simulink model "B733_JSB_R17a"  (R2017a)
settings: Solver=VariableStepAuto  StartTime=0.0  StopTime=simtime  RelTol=1e-3
undefined symbols (not defined in the file): engineCount, engineLUT, Tmil, xu
libraries: aerolibanim x1, aerolibatmos2 x1, aerolibgravity2 x1
settings Model: Creator=Can Bekar  LastModifiedBy=Can Bekar
settings DataIOCC: ExternalInput=usignal  InitialState=xu  LoadExternalInput=on  LoadInitialState=on  SaveFormat=Array

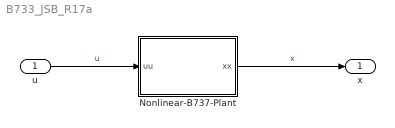
== system B733_JSB_R17a ==
  u : Inport
  Nonlinear-B737-Plant : Subsystem
  x : Outport
  wires:
  u/1 -> Nonlinear-B737-Plant/1(uu)  "u"
  Nonlinear-B737-Plant/1(xx) -> x/1  "x"

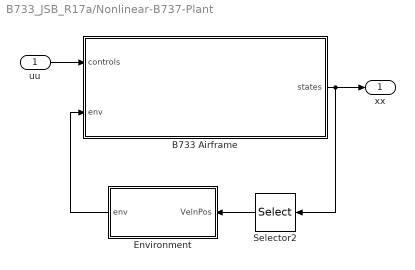
== system B733_JSB_R17a/Nonlinear-B737-Plant ==
  uu : Inport
  B733 Airframe : Subsystem
      mask Display: image('300Large.png');
  Environment : Subsystem
      mask Display: image('ww15mgh2.jpg');
  Selector2 : Selector  InputPortWidth=12  IndexOptions=Index vector (dialog)  Indices=[1 10 11 12]  OutputSizes=1
  xx : Outport
  wires:
  uu/1 -> B733 Airframe/1(controls)
  B733 Airframe/1(states) -> xx/1, Selector2/1
  Selector2/1 -> Environment/1(VelnPos)
  Environment/1(env) -> B733 Airframe/2(env)

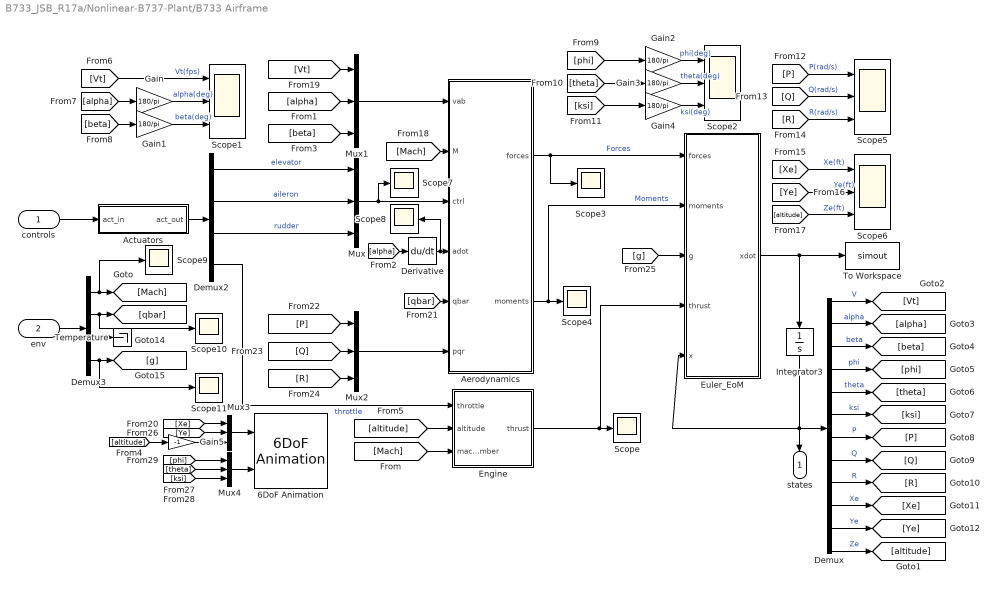
== system B733_JSB_R17a/Nonlinear-B737-Plant/B733 Airframe ==
  controls : Inport
  env : Inport  Port=2
  6DoF Animation : aerolibanim/6DoF Animation  u1=[0 100000 -100000 100000 0 35000]  u2=1  u3=15000.0  u4=[0 0 0]  u5=Fixed position  u6=[100000 20000 -xu(12)]  u7=30  u8=on
      settings: SourceProductName=Aerospace Blockset
  Actuators : Subsystem
  Aerodynamics : MATLAB Function  TreatAsAtomicUnit=on
  Demux : Demux  Outputs=12
  Demux2 : Demux
  Demux3 : Demux
  Derivative : Derivative
  Engine : Subsystem
  Euler_EoM : MATLAB Function  TreatAsAtomicUnit=on
  Gain{,1..4} (5 alike) : Gain  Gain=180/pi
  Gain5 : Gain  Gain=-1
  Integrator3 : Integrator  InitialCondition=xu
  Mux{,1..4} (5 alike) : Mux  Inputs=3
  Scope{,3..4,7..11} (8 alike) : Scope
  Scope{1..2,5..6} (4 alike) : Scope  NumInputPorts=3
  Temperature : Terminator
  To Workspace : ToWorkspace  VariableName=simout  SampleTime=-1
  states : Outport
  wires:
  Actuators/1(act_out) -> Demux2/1
  [Mach] -> Engine/3(mach_number)
  Integrator3/1 -> Euler_EoM/5(x), states/1, Demux/1
  Demux/1 -> [Vt]  "V"
  Demux/3 -> [beta]  "beta"
  [alpha] -> Derivative/1
  [altitude] -> Engine/2(altitude)
  Demux/12 -> [altitude]  "Ze"
  [Vt] -> Scope1/1  "Vt(fps)"
  Demux/11 -> [Ye]  "Ye"
  Demux/10 -> [Xe]  "Xe"
  Demux/9 -> [R]  "R"
  Demux/8 -> [Q]  "Q"
  Demux/7 -> [P]  "P"
  Demux/6 -> [ksi]  "ksi"
  Demux/5 -> [theta]  "theta"
  Demux/4 -> [phi]  "phi"
  [theta] -> Gain3/1
  [phi] -> Gain2/1
  [ksi] -> Gain4/1
  [R] -> Scope5/3  "R(rad/s)"
  [Q] -> Scope5/2  "Q(rad/s)"
  [P] -> Scope5/1  "P(rad/s)"
  [Xe] -> Scope6/1  "Xe(ft)"
  [altitude] -> Scope6/3  "Ze(ft)"
  [Ye] -> Scope6/2  "Ye(ft)"
  Engine/1(thrust) -> Euler_EoM/4(thrust), Scope/1
  [Mach] -> Aerodynamics/2(M)
  Demux2/1 -> Mux/1  "elevator"
  Demux2/2 -> Mux/2  "aileron"
  Demux2/3 -> Mux/3  "rudder"
  [qbar] -> Aerodynamics/5(qbar)
  Gain/1 -> Scope1/2  "alpha(deg)"
  [alpha] -> Gain/1
  [beta] -> Gain1/1
  Gain1/1 -> Scope1/3  "beta(deg)"
  Aerodynamics/1(forces) -> Scope3/1, Euler_EoM/1(forces)  "Forces"
  Aerodynamics/2(moments) -> Euler_EoM/2(moments), Scope4/1  "Moments"
  [g] -> Euler_EoM/3(g)
  Demux/2 -> [alpha]  "alpha"
  Euler_EoM/1(xdot) -> To Workspace/1, Integrator3/1
  Gain2/1 -> Scope2/1  "phi(deg)"
  Gain3/1 -> Scope2/2  "theta(deg)"
  Gain4/1 -> Scope2/3  "ksi(deg)"
  controls/1 -> Actuators/1(act_in)
  Demux2/4 -> Engine/1(throttle)  "throttle"
  env/1 -> Demux3/1
  Demux3/1 -> Scope9/1, [Mach]
  Demux3/2 -> Scope10/1, [qbar]
  Demux3/3 -> Temperature/1
  Demux3/4 -> Scope11/1, [g]
  Mux/1 -> Scope7/1, Aerodynamics/3(ctrl)
  [Vt] -> Mux1/1
  [beta] -> Mux1/3
  [alpha] -> Mux1/2
  Mux1/1 -> Aerodynamics/1(vab)
  [P] -> Mux2/1
  [Q] -> Mux2/2
  [R] -> Mux2/3
  Mux2/1 -> Aerodynamics/6(pqr)
  Mux4/1 -> 6DoF Animation/2
  Mux3/1 -> 6DoF Animation/1
  [Ye] -> Mux3/2
  [Xe] -> Mux3/1
  [ksi] -> Mux4/3
  [phi] -> Mux4/1
  [theta] -> Mux4/2
  [altitude] -> Gain5/1
  Derivative/1 -> Scope8/1, Aerodynamics/4(adot)
  Gain5/1 -> Mux3/3

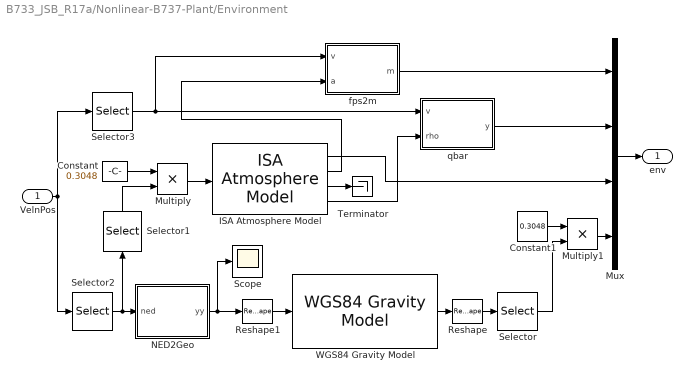
== system B733_JSB_R17a/Nonlinear-B737-Plant/Environment ==
  VelnPos : Inport
  Constant : Constant  Value=0.3048
  Constant1 : Constant  Value=0.3048
  ISA Atmosphere Model : aerolibatmos2/ISA Atmosphere Model  custom=off  g=9.80665  gamma=1.4  R=287.0531  L=0.0065  h_trop=11000  h_strat=20000  rho0=1.225  P0=101325  T0=288.15  h0=0
      settings: SourceProductName=Aerospace Blockset
  Multiply : Product
  Multiply1 : Product
  Mux : Mux
  NED2Geo : MATLAB Function  TreatAsAtomicUnit=on
  Reshape : Reshape
  Reshape1 : Reshape  OutputDimensionality=Customize  OutputDimensions=[1,3]
  Scope : Scope
  Selector : Selector  InputPortWidth=3  IndexOptions=Index vector (dialog)  Indices=[3]  OutputSizes=1
  Selector1 : Selector  InputPortWidth=3  IndexOptions=Index vector (dialog)  Indices=[3]  OutputSizes=1
  Selector2 : Selector  InputPortWidth=4  IndexOptions=Index vector (dialog)  Indices=[2 3 4]  OutputSizes=1
  Selector3 : Selector  InputPortWidth=4  IndexOptions=Index vector (dialog)  Indices=[1]  OutputSizes=1
  Terminator : Terminator
  "WGS84 Gravity Model  " : aerolibgravity2/WGS84 Gravity Model   units=English
      settings: SourceProductName=Aerospace Blockset  SourceProductBaseCode=AE
  fps2m : MATLAB Function  TreatAsAtomicUnit=on
  qbar : MATLAB Function  TreatAsAtomicUnit=on
  env : Outport
  wires:
  Selector3/1 -> fps2m/1(v), qbar/1(v)
  Mux/1 -> env/1
  Multiply/1 -> ISA Atmosphere Model/1
  Constant/1 -> Multiply/1
  ISA Atmosphere Model/1 -> Mux/3
  ISA Atmosphere Model/2 -> fps2m/2(a)
  ISA Atmosphere Model/3 -> Terminator/1
  fps2m/1(m) -> Mux/1
  ISA Atmosphere Model/4 -> qbar/2(rho)
  qbar/1(y) -> Mux/2
  Multiply1/1 -> Mux/4
  Constant1/1 -> Multiply1/1
  "WGS84 Gravity Model  "/1 -> Reshape/1
  Reshape/1 -> Selector/1
  Selector/1 -> Multiply1/2
  Reshape1/1 -> "WGS84 Gravity Model  "/1
  NED2Geo/1(yy) -> Scope/1, Reshape1/1
  VelnPos/1 -> Selector2/1, Selector3/1
  Selector1/1 -> Multiply/2
  Selector2/1 -> Selector1/1, NED2Geo/1(ned)

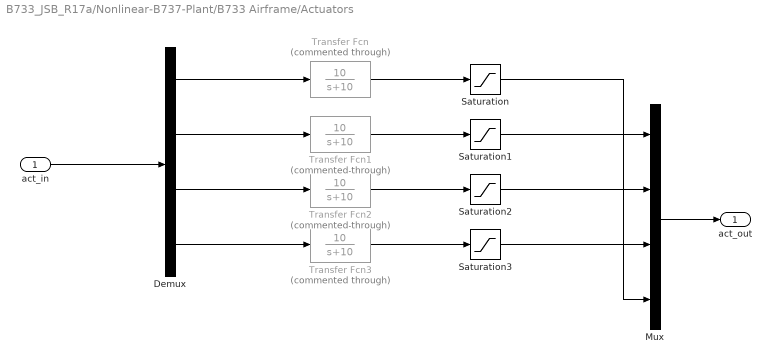
== system B733_JSB_R17a/Nonlinear-B737-Plant/B733 Airframe/Actuators ==
  act_in : Inport
  Demux : Demux
  Mux : Mux
  Saturation : Saturate  UpperLimit=1  LowerLimit=0  OutMin=[0]  OutMax=[1]
  Saturation1 : Saturate  UpperLimit=0.3  LowerLimit=-0.3  OutMin=[-0.3]  OutMax=[0.3]
  Saturation2 : Saturate  UpperLimit=0.35  LowerLimit=-0.35  OutMin=[-0.35]  OutMax=[0.35]
  Saturation3 : Saturate  UpperLimit=0.35  LowerLimit=-0.35  OutMin=[-0.35]  OutMax=[0.35]
  Transfer Fcn : TransferFcn  Commented=through  Numerator=[10]  Denominator=[1 10]  ContinuousStateAttributes='throttle'
  Transfer Fcn1 : TransferFcn  Commented=through  Numerator=[10]  Denominator=[1 10]  ContinuousStateAttributes='elevator_deflection'
  Transfer Fcn2 : TransferFcn  Commented=through  Numerator=[10]  Denominator=[1 10]  ContinuousStateAttributes='Aileron_deflection'
  Transfer Fcn3 : TransferFcn  Commented=through  Numerator=[10]  Denominator=[1 10]  ContinuousStateAttributes='Rudder_deflection'
  act_out : Outport
  wires:
  act_in/1 -> Demux/1
  Demux/1 -> Transfer Fcn/1
  Demux/2 -> Transfer Fcn1/1
  Demux/3 -> Transfer Fcn2/1
  Demux/4 -> Transfer Fcn3/1
  Transfer Fcn/1 -> Saturation/1
  Transfer Fcn1/1 -> Saturation1/1
  Transfer Fcn2/1 -> Saturation2/1
  Transfer Fcn3/1 -> Saturation3/1
  Mux/1 -> act_out/1
  Saturation1/1 -> Mux/1
  Saturation2/1 -> Mux/2
  Saturation3/1 -> Mux/3
  Saturation/1 -> Mux/4

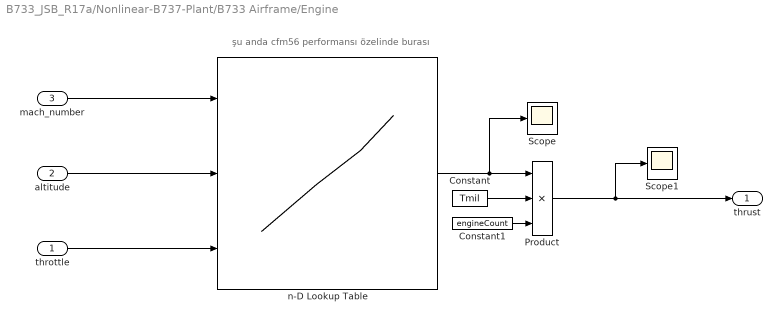
== system B733_JSB_R17a/Nonlinear-B737-Plant/B733 Airframe/Engine ==
  note: şu anda cfm56 performansı özelinde burası
  throttle : Inport
  altitude : Inport  Port=2
  mach_number : Inport  Port=3
  Constant : Constant  Value=Tmil
  Constant1 : Constant  Value=engineCount
  Product : Product  Inputs=3
  Scope : Scope
  Scope1 : Scope
  n-D Lookup Table : Lookup_n-D  NumberOfTableDimensions=3  BreakpointsSpecification=Even spacing  BreakpointsForDimension1=[0]  BreakpointsForDimension2=[]  BreakpointsForDimension3=[]  BreakpointsForDimension1FirstPoint=0  BreakpointsForDimension2FirstPoint=-10000  BreakpointsForDimension3FirstPoint=0  BreakpointsForDimension1Spacing=0.2  BreakpointsForDimension2Spacing=10000  Table=engineLUT  InternalRulePriority=Speed  RndMeth=Simplest  InputSameDT=on
  thrust : Outport
  wires:
  altitude/1 -> n-D Lookup Table/2
  n-D Lookup Table/1 -> Scope/1, Product/1
  mach_number/1 -> n-D Lookup Table/1
  throttle/1 -> n-D Lookup Table/3
  Constant/1 -> Product/2
  Constant1/1 -> Product/3
  Product/1 -> Scope1/1, thrust/1

== matlab function B733_JSB_R17a/Nonlinear-B737-Plant/Environment/NED2Geo ==
  data: ned input; yy output
function yy = fcn(ned)
yy = [0,0,0];
coder.extrinsic('ned2geodetic'); 
coder.extrinsic('wgs84Ellipsoid'); 
ellipsoid = wgs84Ellipsoid;
[lat,lon,h] = ned2geodetic(ned(1),ned(2),-ned(3),40.976111, 28.814167,0,ellipsoid);
yy = [lat,lon,h];
end

== matlab function B733_JSB_R17a/Nonlinear-B737-Plant/B733 Airframe/Euler_EoM ==
  data: forces input; moments input; g input; xdot output; thrust input; x input
function xdot = Zeom_fcn(forces,moments, g, thrust,x)

xdot = zeros(12,1);

%TODO fuel to be added
weight = 83000; %Weight of Aircraft (lb)
gd     = g*3.28084; %Gravitational Acceleration
m      = weight/gd; %Mass(slug)

Heng  = 0;

Jxx = 562000;
Jyy = 1.473e+06;
Jzz = 1.894e+06;
Jxz = 8000;

Vt    = x(1);
alpha = x(2);
beta  = x(3);
phi   = x(4);
theta = x(5);
ksi   = x(6);
P     = x(7);
Q     = x(8);
R     = x(9);

T   = thrust;

Fx = forces(1); %CD
Fy = forces(2); %CL
Fz = forces(3); %CC

L = moments(1); %Cl
M = moments(2); %Cm
N = moments(3); %Cn

cp = cos(phi);
ct = cos(theta);
ck = cos(ksi);
sp = sin(phi);
st = sin(theta);
sk = sin(ksi);
tt = tan(theta);

%**************FORCE EQUATIONS**************%  

U = Vt * cos(alpha)*cos(beta);
V = Vt * sin(beta);
W = Vt * sin(alpha)*cos(beta);

UDOT  = R*V  - Q*W - gd*st + (Fx + T)/m; 
VDOT  = P*W  - R*U + gd*sp*ct + Fy/m;
WDOT  = Q*U  - P*V + gd*cp*ct + Fz/m;

xdot(1) = (U*UDOT + V*VDOT + W*WDOT)/Vt;     %Vtdot
xdot(2) = (U*WDOT - W*UDOT)/(U*U + W*W);     %alphadot
xdot(3) = (Vt*VDOT- V*xdot(1))/(U*U + W*W);  %betadot

%**************KINEMATIC EQUATIONS**************%

xdot(4) = P + tt*(Q*sp + R*cp); %phidot
xdot(5) = Q*cp - R*sp;          %thetadot
xdot(6) = Q*sp/ct + R*cp/ct;    %ksidot

%**************MOMENT EQUATIONS**************%

xdot(7) = (Jxz*(Jxx-Jyy+Jzz)*P*Q - (Jzz*(Jzz-Jyy)+Jxz^2)*Q*R + Jzz*L + Jxz*(N + Q*Heng))/(Jxx*Jzz-Jxz^2);  %pdot
xdot(8) = ((Jzz-Jxx)*P*R - Jxz*(P^2 - R^2) + M - R*Heng )/Jyy; %qdot
xdot(9) = (((Jxx-Jyy)*Jxx+Jxz^2)*P*Q - Jxz*(Jxx-Jyy+Jzz)*Q*R + Jxz*L + Jxx*(N + Q*Heng))/(Jxx*Jzz-Jxz^2);  %rdot

%**************NAVIGATION EQUATIONS**************%

xdot(10) = U*ct*ck + V*(-cp*sk + sp*st*ck) + W*(sp*sk + cp*st*ck);  %xdot
xdot(11) = U*ct*sk + V*(cp*ck + sp*st*sk) + W*(-sp*ck + cp*st*sk);  %ydot
xdot(12) = U*st - V*sp*ct - W*cp*ct;                                %altdot
end

== matlab function B733_JSB_R17a/Nonlinear-B737-Plant/Environment/fps2m ==
  data: v input; m output; a input
function m = fps2m(v,a)
m= v/(a*3.28084);
end

== matlab function B733_JSB_R17a/Nonlinear-B737-Plant/Environment/qbar ==
  data: v input; rho input; y output
function y = qbar(v, rho)
y = 0.5*rho*v*v*0.0019577143;

== matlab function B733_JSB_R17a/Nonlinear-B737-Plant/B733 Airframe/Aerodynamics ==
  data: vab input; M input; ctrl input; adot input; qbar input; pqr input; forces output; moments output
function [forces, moments] = aeromodel(vab, M, ctrl,  adot, qbar, pqr)
forces = zeros(1,3);
moments = zeros(1,3);
coder.extrinsic('Zaero_fn'); 
[forces, moments] = Zaero_fn(vab(1), M, ctrl(1), ctrl(2), ctrl(3), vab(2), vab(3), adot, qbar, pqr(1), pqr(2), pqr(3));
end
